simulink model "mcb_pmsm_param_est_MCSPTE1AK144"  (R2023a)
settings: Solver=FixedStepDiscrete  StartTime=0.0  StopTime=6  RelTol=1e-3  EnableMultiTasking=on
PreLoadFcn:
  | mcb_pmsm_param_est_MCSPTE1AK144_data;
InitFcn:
  | mbd_s32k_consistency_checks(bdroot(gcs));
undefined symbols (not defined in the file): External, inverter, LQFP, motor, One, Shot, TRGMUX_PDB_TRIG, Ts, Ts_uart
libraries: mbd_s32k1xx_ec_toolbox x30, simulink x6, mbd_msd_ec_toolbox x4, mcbpmsmparamestlib x4, embeddedblockslib x1
Description:
  | Open Loop Loop Control of 3-phase motor with MTRDEVSPNK144.
  | This Simulink model is designed to work with Linix 45ZWN24-40 Motor and validate
  | that the motor can be rotated in open loop using Mathworks model from Motor Control Blockset.
  | The main scope of the model is to validate the 3-phase current measurements.
  | 
  | FEATURES:
  | - Alternatively, use FreeMASTER pannel to control the speed and direction
  | - Measure the 3-phase sinusoidal currents with PWM-PDB-ADC synchronization
  | - Measure the DC bus voltage and current with PWM-PDB-ADC synchronization
  | 
  | HW SETUP:
  | - Configure S32K144 board supply voltage: J107:2-3(over USB)
  | - Configure J9,J10 and J11 on MotorGD: 2-3 (mode PMSM)
  | - Rotate trimmer resistor R72 (placed Devkit-MotorGD) counter-clockwise at maximum
  | - Power on the kit via J7 connector with 12Vdc
  | 
  | VALIDATION:
  | - First run 'mcb_open_loop_control_data_MTRDEVKSPNK144.m' file to load parameters in workspace,
  | - Build/Simulate the model,
  | - After reset or power on, the Green LED shall be ON
  | - In case of a FAULT the Red LED will be ON
  | - Open FreeMASTER project and connect to the target.
  | - Click on "App" tab and set the desired motor speed then click on the ON/OFF button
  | 
  | NOTE:
  | - In case of fault (RED LED is ON), the remove fault cause and press RESET button
  | 
  | Copyright (c) 2020 NXP
  | version 1.0.0
settings Model: Creator=NXP MBDT Team  LastModifiedBy=snarayan
settings SolverCC: AlgebraicLoopSolver=TrustRegion  AutoInsertRateTranBlk=on
settings DataIOCC: ExternalInput=off  InitialState=off  SaveFormat=Array  SaveOutput=off  SaveTime=off  ReturnWorkspaceOutputs=off
settings OptimizationCC: DefaultParameterBehavior=Inlined  UseFloatMulNetSlope=on  DefaultUnderspecifiedDataType=single  UseSpecifiedMinMax=on  EnhancedBackFolding=on  PassReuseOutputArgsAs=Individual arguments  ZeroExternalMemoryAtStartup=off  ZeroInternalMemoryAtStartup=off  NoFixptDivByZeroProtection=on  EfficientFloat2IntCast=on  OptimizeBlockOrder=speed  DifferentSizesBufferReuse=on  EfficientTunableParamExpr=on
settings DebuggingCC: CheckSSInitialOutputMsg=off  UnderspecifiedInitializationDetection=Classic  MergeDetectMultiDrivingBlocksExec=none  SolverPrmCheckMsg=warning  InheritedTsInSrcMsg=none  MultiTaskDSMMsg=none  SingleTaskRateTransMsg=error  ParameterPrecisionLossMsg=none  ParameterTunabilityLossMsg=error  UnconnectedInputMsg=error  UnconnectedOutputMsg=error  UnconnectedLineMsg=error  AssertControl=DisableAll  AllowSymbolicDim=off  UnknownTsInhSupMsg=error  StateNameClashWarn=warning  SFUnexpectedBacktrackingDiag=warning  SFNoUnconditionalDefaultTransitionDiag=warning  SFExecutionAtInitializationDiag=none  ArithmeticOperatorsInVariantConditions=warning
settings HardwareCC: ProdBitPerPointer=32  ProdBitPerSizeT=32  ProdBitPerPtrDiffT=32  ProdLargestAtomicInteger=Long  ProdLargestAtomicFloat=Double  ProdWordSize=32  ProdHWDeviceType=ARM Compatible->ARM Cortex
settings ModelReferenceCC: EnableRefExpFcnMdlSchedulingChecks=on
settings SFSimCC: SimUseLocalCustomCode=off  MATLABDynamicMemAlloc=off  CustomCodeUndefinedFunction=UseInterfaceOnly
settings RTWCC: Description=Model Based Design Toolbox S32K1xx Code Generation Target  SystemTargetFile=mbd_s32k.tlc  MakeCommand=mbd_s32k_make_rtw COPY_MDLREF_INCLUDES=0  TemplateMakefile=mbd_s32k.tmf  RTWUseLocalCustomCode=off  IncludeHyperlinkInReport=on  DLArmComputeVersion=19.05
settings CodeAppCC: ForceParamTrailComments=on  IgnoreCustomStorageClasses=off  MaxIdLength=64  OperatorAnnotations=on  SimulinkDataObjDesc=on  SFDataObjDesc=on  InsertBlockDesc=on  InternalIdentifier=Classic
settings STFCustomTargetCC: MultiwordLength=256  ConcurrentExecutionCompliant=off  CombineOutputUpdateFcns=on  ERTCustomFileBanners=on  SupportContinuousTime=off  SupportNonInlinedSFcns=off  RemoveResetFunc=on  MATLABClassNameForMDSCustomization=Simulink.SoftwareTarget.ERTCustomization  GRTInterface=off  UseToolchainInfoCompliant=off  SystemTargetFile=mbd_s32k.tlc
settings ERTTargetCC: TargetLangStandard=C99 (ISO)  ParMdlRefBuildCompliant=off  CompOptLevelCompliant=off  ConcurrentExecutionCompliant=off  ModelStepFunctionPrototypeControlCompliant=off  CPPClassGenCompliant=off  UseToolchainInfoCompliant=off  InlinedParameterPlacement=NonHierarchical  ERTSrcFileBannerTemplate=mbd_ert_code_template.cgt  ERTHdrFileBannerTemplate=mbd_ert_code_template.cgt  ERTDataSrcFileTemplate=mbd_ert_code_template.cgt  ERTDataHdrFileTemplate=mbd_ert_code_template.cgt  ERTCustomFileTemplate=example_file_process.tlc
settings ConfigComp: CovMetricSettings=dw  CovSaveCumulativeToWorkspaceVar=on  CovSaveSingleToWorkspaceVar=on  CovExternalEMLEnable=off

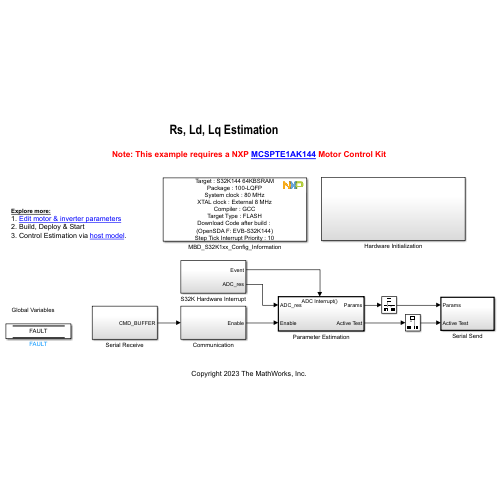
[thumbnail: Simulink's stored preview of the top-level diagram]
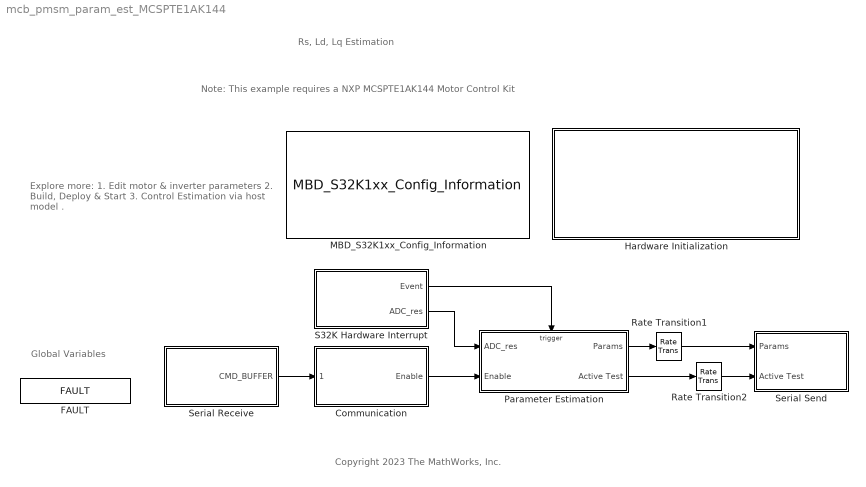
== system mcb_pmsm_param_est_MCSPTE1AK144 ==
  note: Copyright 2023 The MathWorks, Inc.
  note: Rs, Ld, Lq Estimation
  note: Explore more:
      | 1. Edit motor & inverter parameters
      | 2. Build, Deploy & Start
      | 3. Control Estimation via host model .
  note: Note: This example requires a NXP MCSPTE1AK144 Motor Control Kit
  note: Global Variables
  Communication : Subsystem
  FAULT : DataStoreMemory  DataStoreName=FAULT  WriteAfterWriteMsg=warning  WriteAfterReadMsg=warning  ShowAdditionalParam=off  OutDataTypeStr=boolean
  Hardware Initialization : Subsystem  Priority=2
  MBD_S32K1xx_Config_Information : mbd_s32k1xx_ec_toolbox/MBD_S32K1xx_Config_Information  Priority=1  mbdt_ver=0  disp_str=|  config_params=[]  mcu_target_name=S32K144  mcu_target_package=100-LQFP  mcu_target_sram_size=64KB  mcu_system_clock_freq=80  mcu_xtal_freq=External 8  mcu_steptick_timer=LPIT Channel 0  mcu_steptick_prio=10  ds_import_enable=on  target_compiler=GCC  target_memory=FLASH  gcc_target_compile_opts=-mcpu=cortex-m4 -mthumb -mfloat-abi=hard -mfpu=fpv4-sp-d16 -O1 -g -gstrict-dwarf  gcc_target_assemble_opts=-mcpu=cortex-m4 -mthumb -mfloat-abi=hard -mfpu=fpv4-sp-d16 -g  gcc_target_link_opts=-mcpu=cortex-m4 -mthumb -mfloat-abi=hard -mfpu=fpv4-sp-d16  gcc_target_default_lcf=on  gcc_target_user_lcf=S32K144_64_flash.ld  ghs_target_compile_opts=-cpu=cortexm4f -thumb -DARM_MATH_CM4 -fpu=vfpv4_d16 -fsingle -Ogeneral -Wundef -Wimplicit-int -Wshadow -Wtrigraphs --no_commons --gnu_asm -gnu99 -gdwarf-2 -G  ghs_target_assemble_opts=-cpu=cortexm4f -fpu=vfpv4_d16  ghs_target_link_opts=-cpu=cortexm4f -thumb -fpu=vfpv4_d16  ghs_target_default_lcf=on  ghs_target_user_lcf=S32K144_64_flash.ld  iar_target_compile_opts=--cpu=Cortex-M4F --thumb --fpu=VFPv4_sp -Ol -e --debug --dlib_config normal  iar_target_assemble_opts=--cpu Cortex-M4F --thumb --fpu VFPv4_sp  iar_target_link_opts=--no_exceptions --vfe --inline  iar_target_default_lcf=on  iar_target_user_lcf=S32K144_64_flash.icf  pil_download_enable=off  rbl_download_enable=on  rbl_start_delay=5000  rbl_download_interface=OpenSDA  rbl_restart_request=off  rbl_com_port=Custom  rbl_com_port_custom=COM1  pil_download_rate=57600  pil_opensda_drive=F: EVB-S32K144  pil_opensda_drive_custom=D  pil_uart_instance=1  pil_uart_rx=PTC6: [LPUART1_RX | Receive]  pil_uart_tx=PTC7: [LPUART1_TX | Transmit]  FTM_PWM_PcrCheckEnDis=on  FTM_Input_Edge_Inputs_PcrCheckEnDis=on  FTM_Dual_Edge_Inputs_PcrCheckEnDis=on  FTM_Quadrature_Inputs_PcrCheckEnDis=on  FTM_Hall_Sensor_Inputs_PcrCheckEnDis=on  LPTMR_PcrCheckEnDis=on  PIT_PcrCheckEnDis=on  RTC_PcrCheckEnDis=on  FlexCAN_PcrCheckEnDis=on  LIN_PcrCheckEnDis=on  FlexIO_PcrCheckEnDis=on  LPI2C_PcrCheckEnDis=on  LPSPI_PcrCheckEnDis=on  LPUART_PcrCheckEnDis=on  CMP_PcrCheckEnDis=on  GPIO_OutputPcrCheckEnDis=on  GPIO_InputPcrCheckEnDis=on  SBC_PcrCheckEnDis=on  BMS_PcrCheckEnDis=on  AMMCLIB_PcrCheckEnDis=on  FM_PcrCheckEnDis=on  Profile_PcrCheckEnDis=on  ConfigParams_PcrCheckEnDis=on  ModelRef_PcrCheckEnDis=on  PDB0_PcrCheckEnDis=on  CSEc_PcrCheckEnDis=on  eDMA_PcrCheckEnDis=on  FLASH_PcrCheckEnDis=on  ADC_PcrCheckEnDis=on  WDOG_PcrCheckEnDis=on
      | Target : S32K144-64KB_SRAM
      | Package : 100-pin
      | System clock : 80 MHz
      | XTAL clock : External 8 MHz
      | Compiler : IAR
      | Target Type : FLASH
      | Download Code after build : off
      | Step Tick Interrupt Priority : 15
  Parameter Estimation : Subsystem
      settings: RTWSystemCode=Nonreusable function
  Rate Transition1 : RateTransition  Integrity=off  Deterministic=off
  Rate Transition2 : RateTransition  Integrity=off  Deterministic=off
  S32K Hardware Interrupt : Subsystem
  Serial Receive : Subsystem  SystemSampleTime=1e-3
      settings: RTWSystemCode=Nonreusable function
  Serial Send : Subsystem  TreatAsAtomicUnit=on  SystemSampleTime=Ts_uart
  wires:
  Rate Transition1/1 -> Serial Send/1(Params)
  S32K Hardware Interrupt/2(ADC_res) -> Parameter Estimation/1(ADC_res)
  S32K Hardware Interrupt/1(Event) -> Parameter Estimation/Trigger
  Communication/1(Enable) -> Parameter Estimation/2(Enable)
  Serial Receive/1(CMD_BUFFER) -> Communication/1(" ")
  Parameter Estimation/1(Params) -> Rate Transition1/1
  Parameter Estimation/2(Active Test) -> Rate Transition2/1
  Rate Transition2/1 -> Serial Send/2(Active Test)

== system mcb_pmsm_param_est_MCSPTE1AK144/Communication ==
  " " : Inport
  Data Type Conversion : DataTypeConversion  OutDataTypeStr=int16  ConvertRealWorld=Stored Integer (SI)  RndMeth=Simplest  SaturateOnIntegerOverflow=off
  Data Type Conversion3 : DataTypeConversion  OutDataTypeStr=boolean  RndMeth=Simplest  SaturateOnIntegerOverflow=off
  Demux : Demux  Outputs=2
  Rate Transition : RateTransition  Deterministic=off  InitialCondition=[0 0]  OutPortSampleTime=Ts
  Terminator : Terminator
  Enable : Outport  VectorParamsAs1DForOutWhenUnconnected=off
  wires:
  " "/1 -> Rate Transition/1
  Rate Transition/1 -> Demux/1
  Demux/2 -> Data Type Conversion3/1
  Demux/1 -> Data Type Conversion/1
  Data Type Conversion3/1 -> Enable/1
  Data Type Conversion/1 -> Terminator/1

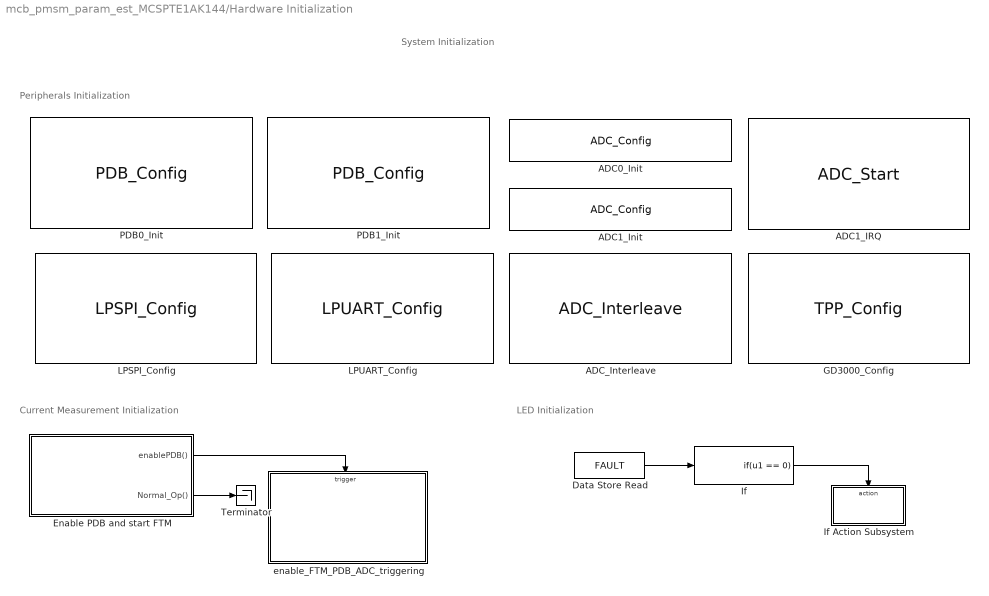
== system mcb_pmsm_param_est_MCSPTE1AK144/Hardware Initialization ==
  note: Peripherals Initialization
  note: System Initialization
  note: Current Measurement Initialization
  note: LED Initialization
  ADC0_Init : mbd_s32k1xx_ec_toolbox/Motor Control Blocks/ADC Blocks/ADC_Config  Priority=3  instance=0  mode=12-bit conversion  smplts=2  adiclk=alternate clock 1  adiv=input clock  show_adv_opts=on  pretrgsel=PDB pre-trigger  swpretrg=Disabled  adtrg=hardware  trgsel=PDB output  refsel=Vrefh and Vrefl  supply_monitoring=off  acfe=off  acfgt=off  acren=off  cv1=0  cv2=0  adco=off  avge=off  avgs=4 samples
  ADC1_IRQ : mbd_s32k1xx_ec_toolbox/Motor Control Blocks/ADC Blocks/ADC_Start  Priority=5  instance=1  adc_r=C  adc_chan=PTB16: [ADC1_SE15 | ADC Single Ended Input]  aien=on  mcuTargetUpdate=on
  ADC1_Init : mbd_s32k1xx_ec_toolbox/Motor Control Blocks/ADC Blocks/ADC_Config  Priority=4  instance=1  mode=12-bit conversion  smplts=2  adiclk=alternate clock 1  adiv=input clock  show_adv_opts=on  pretrgsel=PDB pre-trigger  swpretrg=Disabled  adtrg=hardware  trgsel=PDB output  refsel=Vrefh and Vrefl  supply_monitoring=off  acfe=off  acfgt=off  acren=off  cv1=0  cv2=0  adco=off  avge=off  avgs=4 samples
  ADC_Interleave : mbd_s32k1xx_ec_toolbox/Motor Control Blocks/ADC Blocks/ADC_Interleave  adcInterleavePins=PTB1 to ADC0_SE5 and ADC1_SE15  adcInterleaveInit=on
  Data Store Read : DataStoreRead  DataStoreName=FAULT  IndexOptions=Index vector (dialog)  Indices=1  OutputSizes=1
  Enable PDB and start FTM : Stateflow chart  TreatAsAtomicUnit=on
  GD3000_Config : mbd_msd_ec_toolbox/TPP/TPP_Config  Priority=1  tppInstance=0  desatMode=on  fullonMode=off  lockMode=off  overtempEvent=on  phaseEvent=off  desatEvent=off  framingEvent=on  vlsEvent=on  writeErrEvent=on  overcurrentEvent=on  resetEvent=on  mcuTppIntEn=off  prioInt=15  tppDeadtime=500  initTppNow=on  tppSpiInst=0  tppPwmModule=3  tppPair0_1=on  tppPair2_3=on  tppPair4_5=on  tppPair6_7=off  tppFirstChHS=on  tppEn1Pin=PTA2: [PTA2 | Port A I/O]  tppEn2Pin=PTA2: [PTA2 | Port A I/O]  tppRstPin=PTA3: [PTA3 | Port A I/O]  tppCsPin=PTB5: [PTB5 | Port B I/O]  tppIntPin=PTE10: [PTE10 | Port E I/O]
  If : If  IfExpression=u1 == 0  ShowElse=off
  If Action Subsystem : Subsystem  TreatAsAtomicUnit=on
  "LPSPI_Config " : mbd_s32k1xx_ec_toolbox/Communication Blocks/SPI Blocks/LPSPI_Config   InstanceNumber=0  Role=Master  BaudRate=2000000  ShowAdvanced=on  sin=PTB3: [LPSPI0_SIN | LPSPI Serial Data Input]  sout=PTB4: [LPSPI0_SOUT | LPSPI Serial Data Output]  sck=PTB2: [LPSPI0_SCK | LPSPI Serial Clock I/O]  pcs0=None  pcs1=PTB5: [LPSPI0_PCS1 | Peripheral Chip Select 1]  pcs2=None  pcs3=None  CPHA=1  CPOL=0  BitOrder=MSB first  TransferSize=8  WhichPCS=0  PCSPol=ActiveLow  ContinuousTransfer=off
  LPUART_Config : mbd_s32k1xx_ec_toolbox/Communication Blocks/UART Blocks/LPUART_Config  Priority=1  instance=1  baudrate=256000  databits=8  parity=None  sbns=1  bothedge=rising edge  rxinv=off  txinv=off  show_adv_opts=on  brk13=13 - 16 bit times  lbkde=13 - 16 bit times  rx=PTC6: [LPUART1_RX | Receive]  tx=PTC7: [LPUART1_TX | Transmit]  cts=PTA6: [LPUART1_CTS | Clear To Send (bar)]  rts=PTA7: [LPUART1_RTS | Request To Send]
  PDB0_Init : mbd_s32k1xx_ec_toolbox/Motor Control Blocks/PDB Blocks/PDB_Config  Priority=1  pdbModule=0  regScCont=One-Shot  regScTrgsel=External (TRGMUX_PDB_TRIG)  trgMuxSel=FTM3 Initialize Trigger  trgMuxSelPin=PTB5: [TRGMUX_IN0 | Trigger Mux Input]  regModModulus=5000  regScPrescaler=1  regScMult=1  regPoenPoen0=off  regPo0DlyDly1=0  regPo0DlyDly2=0  enable_pdb_init=off  show_adv_opts=on  regCh0C1En0=on  regCh0C1En1=off  regCh0C1En2=off  regCh0C1En3=off  regCh0C1En4=off  regCh0C1En5=off  regCh0C1En6=off  regCh0C1En7=off  regCh0C1Bb0=off  regCh0C1Bb1=off  regCh0C1Bb2=off  regCh0C1Bb3=off  regCh0C1Bb4=off  regCh0C1Bb5=off  regCh0C1Bb6=off  regCh0C1Bb7=off  regCh0C1Tos0=Pre-trigger is in delay mode  regCh0C1Tos1=Pre-trigger is in delay mode  regCh0C1Tos2=Pre-trigger is in delay mode  regCh0C1Tos3=Pre-trigger is in delay mode  regCh0C1Tos4=Pre-trigger is in delay mode  regCh0C1Tos5=Pre-trigger is in delay mode  regCh0C1Tos6=Pre-trigger is in delay mode  regCh0C1Tos7=Pre-trigger is in delay mode  regCh0DlyDly0=2000  regCh0DlyDly1=0  regCh0DlyDly2=0  regCh0DlyDly3=0  regCh0DlyDly4=0  regCh0DlyDly5=0  regCh0DlyDly6=0  regCh0DlyDly7=0  regCh1C1En0=off  regCh1C1En1=off  regCh1C1En2=off  regCh1C1En3=off  regCh1C1En4=off  regCh1C1En5=off  regCh1C1En6=off  regCh1C1En7=off  regCh1C1Bb0=off  regCh1C1Bb1=off  regCh1C1Bb2=off  regCh1C1Bb3=off  regCh1C1Bb4=off  regCh1C1Bb5=off  regCh1C1Bb6=off  regCh1C1Bb7=off  regCh1C1Tos0=Pre-trigger is in delay mode  regCh1C1Tos1=Pre-trigger is in delay mode  regCh1C1Tos2=Pre-trigger is in delay mode  regCh1C1Tos3=Pre-trigger is in delay mode  regCh1C1Tos4=Pre-trigger is in delay mode  regCh1C1Tos5=Pre-trigger is in delay mode  regCh1C1Tos6=Pre-trigger is in delay mode  regCh1C1Tos7=Pre-trigger is in delay mode  regCh1DlyDly0=0  regCh1DlyDly1=0  regCh1DlyDly2=0  regCh1DlyDly3=0  regCh1DlyDly4=0  regCh1DlyDly5=0  regCh1DlyDly6=0  regCh1DlyDly7=0
  PDB1_Init : mbd_s32k1xx_ec_toolbox/Motor Control Blocks/PDB Blocks/PDB_Config  Priority=2  pdbModule=1  regScCont=One-Shot  regScTrgsel=External (TRGMUX_PDB_TRIG)  trgMuxSel=FTM3 Initialize Trigger  trgMuxSelPin=PTB5: [TRGMUX_IN0 | Trigger Mux Input]  regModModulus=5000  regScPrescaler=1  regScMult=1  regPoenPoen0=off  regPo0DlyDly1=0  regPo0DlyDly2=0  enable_pdb_init=off  show_adv_opts=on  regCh0C1En0=on  regCh0C1En1=on  regCh0C1En2=on  regCh0C1En3=off  regCh0C1En4=off  regCh0C1En5=off  regCh0C1En6=off  regCh0C1En7=off  regCh0C1Bb0=off  regCh0C1Bb1=off  regCh0C1Bb2=off  regCh0C1Bb3=off  regCh0C1Bb4=off  regCh0C1Bb5=off  regCh0C1Bb6=off  regCh0C1Bb7=off  regCh0C1Tos0=Pre-trigger is in delay mode  regCh0C1Tos1=Pre-trigger is in delay mode  regCh0C1Tos2=Pre-trigger is in delay mode  regCh0C1Tos3=Pre-trigger is in delay mode  regCh0C1Tos4=Pre-trigger is in delay mode  regCh0C1Tos5=Pre-trigger is in delay mode  regCh0C1Tos6=Pre-trigger is in delay mode  regCh0C1Tos7=Pre-trigger is in delay mode  regCh0DlyDly0=0  regCh0DlyDly1=1000  regCh0DlyDly2=2000  regCh0DlyDly3=0  regCh0DlyDly4=0  regCh0DlyDly5=0  regCh0DlyDly6=0  regCh0DlyDly7=0  regCh1C1En0=off  regCh1C1En1=off  regCh1C1En2=off  regCh1C1En3=off  regCh1C1En4=off  regCh1C1En5=off  regCh1C1En6=off  regCh1C1En7=off  regCh1C1Bb0=off  regCh1C1Bb1=off  regCh1C1Bb2=off  regCh1C1Bb3=off  regCh1C1Bb4=off  regCh1C1Bb5=off  regCh1C1Bb6=off  regCh1C1Bb7=off  regCh1C1Tos0=Pre-trigger is in delay mode  regCh1C1Tos1=Pre-trigger is in delay mode  regCh1C1Tos2=Pre-trigger is in delay mode  regCh1C1Tos3=Pre-trigger is in delay mode  regCh1C1Tos4=Pre-trigger is in delay mode  regCh1C1Tos5=Pre-trigger is in delay mode  regCh1C1Tos6=Pre-trigger is in delay mode  regCh1C1Tos7=Pre-trigger is in delay mode  regCh1DlyDly0=0  regCh1DlyDly1=0  regCh1DlyDly2=0  regCh1DlyDly3=0  regCh1DlyDly4=0  regCh1DlyDly5=0  regCh1DlyDly6=0  regCh1DlyDly7=0
  Terminator : Terminator
  enable_FTM_PDB_ADC_triggering : Subsystem  TreatAsAtomicUnit=on
      settings: RTWSystemCode=Inline
  wires:
  Enable PDB and start FTM/1(enablePDB()) -> enable_FTM_PDB_ADC_triggering/Trigger
  Enable PDB and start FTM/2(Normal_Op()) -> Terminator/1
  Data Store Read/1 -> If/1
  If/1 -> If Action Subsystem/Action

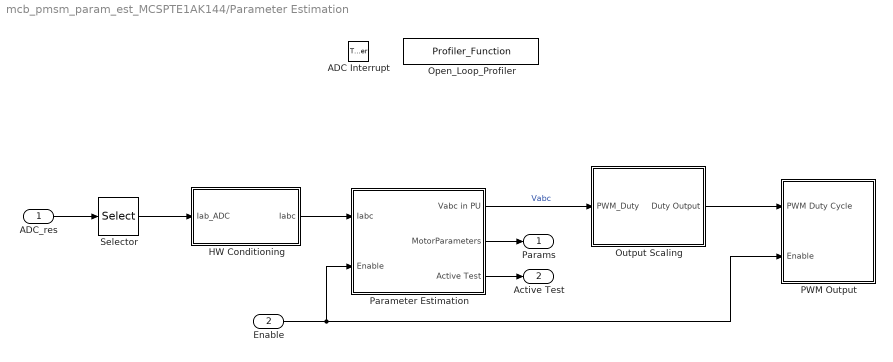
== system mcb_pmsm_param_est_MCSPTE1AK144/Parameter Estimation ==
  ADC_res : Inport
  Enable : Inport  Port=2
  ADC Interrupt : TriggerPort  TriggerType=function-call  VariantControl=Variant
  HW Conditioning : Subsystem
  Open_Loop_Profiler : mbd_s32k1xx_ec_toolbox/Utility Blocks/Profiler_Function  profile_indx=1
  Output Scaling : Subsystem
  PWM Output : Subsystem
  Parameter Estimation : Subsystem
  Selector : Selector  InputPortWidth=4  IndexOptions=Index vector (dialog)  Indices=[1 2]  OutputSizes=1
  Params : Outport
  Active Test : Outport  Port=2
  wires:
  ADC_res/1 -> Selector/1
  Parameter Estimation/1(Vabc in PU) -> Output Scaling/1(PWM_Duty)  "Vabc"
  Output Scaling/1(Duty Output) -> PWM Output/1(PWM Duty Cycle)
  Enable/1 -> Parameter Estimation/2(Enable), PWM Output/2(Enable)
  Parameter Estimation/2(MotorParameters) -> Params/1
  HW Conditioning/1(Iabc) -> Parameter Estimation/1(Iabc)
  Selector/1 -> HW Conditioning/1(Iab_ADC)
  Parameter Estimation/3(Active Test) -> Active Test/1

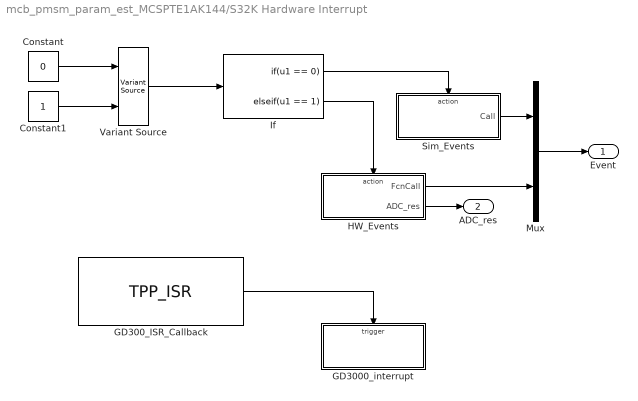
== system mcb_pmsm_param_est_MCSPTE1AK144/S32K Hardware Interrupt ==
  Constant : Constant  Value=0  OutDataTypeStr=Inherit: Inherit via back propagation  SampleTime=-1
  Constant1 : Constant  OutDataTypeStr=Inherit: Inherit via back propagation  SampleTime=-1
  GD3000_interrupt : Subsystem  TreatAsAtomicUnit=on
  "GD300_ISR_Callback " : mbd_msd_ec_toolbox/TPP/TPP_ISR  tppInstance=0
  HW_Events : Subsystem  TreatAsAtomicUnit=on
  If : If  IfExpression=u1 == 0  ElseIfExpressions=u1 == 1  ShowElse=off
  Mux : Mux  Inputs=2
  Sim_Events : Subsystem  TreatAsAtomicUnit=on
  Variant Source : VariantSource  VariantControlMode=sim codegen switching
  Event : Outport
  ADC_res : Outport  Port=2
  wires:
  Constant/1 -> Variant Source/1
  Constant1/1 -> Variant Source/2
  If/2 -> HW_Events/Action
  If/1 -> Sim_Events/Action
  Variant Source/1 -> If/1
  Sim_Events/1(Call) -> Mux/1
  HW_Events/1(FcnCall) -> Mux/2
  Mux/1 -> Event/1
  "GD300_ISR_Callback "/1 -> GD3000_interrupt/Trigger
  HW_Events/2(ADC_res) -> ADC_res/1

== system mcb_pmsm_param_est_MCSPTE1AK144/Serial Receive ==
  Codegen : Subsystem
  Sim : Subsystem
  Variant Source : VariantSource  VariantControlMode=sim codegen switching
  CMD_BUFFER : Outport  InitialOutput=[16384 0]  VectorParamsAs1DForOutWhenUnconnected=off
  wires:
  Sim/1(Out1) -> Variant Source/2
  Variant Source/1 -> CMD_BUFFER/1
  Codegen/1(Out1) -> Variant Source/1

== system mcb_pmsm_param_est_MCSPTE1AK144/Serial Send ==
  Params : Inport
  Active Test : Inport  Port=2
  Demux : Demux  Outputs=3
  LPUART_Transmit : mbd_s32k1xx_ec_toolbox/Communication Blocks/UART Blocks/LPUART_Transmit  Priority=2  instance=1
  Multiport Switch : MultiPortSwitch  DiagnosticForDefault=Warning  OutDataTypeStr=dataType  RndMeth=Simplest  SaturateOnIntegerOverflow=off  InputSameDT=off
  Protocol Encoder : embeddedblockslib/Protocol Encoder  Header='S'  FieldTable={ 'Count', '1', 'uint8', 'Little endian'; 'Parameter', '1', 'single', 'Little endian'; 'Active Test', '1', 'uint8', 'Little endian' }  IsChecksumRequired=off  ChecksumAlgorithm=XOR of bytes  ChecksumSize=[]  TerminatorOption=<none>  CustomTerminatorVal=[]
      settings: LibrarySourceBlock=c2000lib/Target Communication/Protocol Encoder
  Reshape : Reshape
  count to 3 : Subsystem
  wires:
  Protocol Encoder/1 -> Reshape/1
  Reshape/1 -> LPUART_Transmit/1
  Multiport Switch/1 -> Protocol Encoder/2
  Params/1 -> Demux/1
  Demux/1 -> Multiport Switch/2
  Demux/2 -> Multiport Switch/3
  Demux/3 -> Multiport Switch/4
  count to 3/1(count) -> Multiport Switch/1, Protocol Encoder/1
  Active Test/1 -> Protocol Encoder/3

== system mcb_pmsm_param_est_MCSPTE1AK144/Hardware Initialization/If Action Subsystem ==
  Action Port : ActionPort  ActionPortLabel=if(u1 == 0)
  LED_GREEN : Constant  Value=0  OutDataTypeStr=boolean  SampleTime=-1
  LED_GREEN_ON : mbd_s32k1xx_ec_toolbox/GPIO Blocks/Digital_Output  gpio_pin=PTD16: [PTD16 | Port D I/O]  init_val=Low  drive_strength=Low
  LED_RED : Constant  OutDataTypeStr=boolean  SampleTime=-1
  LED_RED_OFF : mbd_s32k1xx_ec_toolbox/GPIO Blocks/Digital_Output  gpio_pin=PTD15: [PTD15 | Port D I/O]  init_val=Low  drive_strength=Low
  wires:
  LED_GREEN/1 -> LED_GREEN_ON/1
  LED_RED/1 -> LED_RED_OFF/1

== system mcb_pmsm_param_est_MCSPTE1AK144/Hardware Initialization/enable_FTM_PDB_ADC_triggering ==
  function : TriggerPort  TriggerType=function-call  VariantControl=(inherit)
  Custom code to reload the PDB value : Subsystem  Priority=6  mask(System Outputs){ShowInLibBrowser=0}
      mask prompts: ShowInLibBrowser "Simulink:masks:CustCodeMaskParam1_MP"
      settings: CopyFcn=cccopyfcn(gcb)  OpenFcn=ccopenfcn('System Outputs Function')
      mask Help: eval('feval(''rtwprivate'',''rtwhelpview'',''rtw_sys_outputs_block'')');
      mask Display: disp('System\nOutputs');
  FTM_Init_Trigger_Disable_Enable : mbd_s32k1xx_ec_toolbox/Motor Control Blocks/FTM Blocks/FTM_Init_Trigger_Disable_Enable  Priority=3  ftmModule=3  action=Enable
  FTM_PWM_Disable_Enable : mbd_s32k1xx_ec_toolbox/Motor Control Blocks/FTM Blocks/FTM_PWM_Disable_Enable  Priority=1  ftmModule=3  action=Enable
  PDB0_Enable : mbd_s32k1xx_ec_toolbox/Motor Control Blocks/PDB Blocks/PDB_Enable  Priority=4  pdbModule=0  pdbAction=Enable
  PDB1_Enable : mbd_s32k1xx_ec_toolbox/Motor Control Blocks/PDB Blocks/PDB_Enable  Priority=5  pdbModule=1  pdbAction=Enable
  TPP_ISR_Enable_Disable : mbd_msd_ec_toolbox/TPP/TPP_ISR_Enable_Disable  Priority=7  tppInstance=0  mcuTppIntEn=on  prioInt=15

== system mcb_pmsm_param_est_MCSPTE1AK144/Parameter Estimation/HW Conditioning ==
  Iab_ADC : Inport
  Add : Sum  Inputs=+-  RndMeth=Simplest  OutDataTypeStr=Inherit: Same as first input
  Constant2 : Constant  Value=0  OutDataTypeStr=single
  Data Type Conversion : DataTypeConversion  OutDataTypeStr=single  RndMeth=Simplest  SaturateOnIntegerOverflow=off
  Gain : Gain  Gain=-inverter.ISenseMax/2048  RndMeth=Simplest  OutDataTypeStr=Inherit: Same as input
  Iab Offset : Constant  Value=[inverter.CtSensAOffset inverter.CtSensBOffset]  OutDataTypeStr=int32
  Mux : Mux  Inputs=2
  Iabc : Outport
  wires:
  Add/1 -> Gain/1
  Data Type Conversion/1 -> Add/1
  Iab_ADC/1 -> Data Type Conversion/1
  Iab Offset/1 -> Add/2
  Constant2/1 -> Mux/2
  Mux/1 -> Iabc/1
  Gain/1 -> Mux/1

== system mcb_pmsm_param_est_MCSPTE1AK144/Parameter Estimation/Output Scaling ==
  PWM_Duty : Inport
  Constant : Constant  OutDataTypeStr=dataType
  Gain : Gain  Gain=0.5  RndMeth=Simplest  OutDataTypeStr=Inherit: Same as input
  Sum : Sum  Inputs=|++  RndMeth=Simplest  OutDataTypeStr=Inherit: Same as first input
  Duty Output : Outport
  wires:
  Gain/1 -> Duty Output/1
  PWM_Duty/1 -> Sum/1
  Constant/1 -> Sum/2
  Sum/1 -> Gain/1

== system mcb_pmsm_param_est_MCSPTE1AK144/Parameter Estimation/PWM Output ==
  PWM Duty Cycle : Inport
  Enable : Inport  Port=2
  Demux : Demux  Outputs=3
  FTM_PWM_Config : mbd_s32k1xx_ec_toolbox/Motor Control Blocks/FTM Blocks/FTM_PWM_Config  ftmModule=3  ftmMode=Center-Aligned PWM  ftmSourceClock=80 MHz  swcontrol_enable=off  chan0En=on  chan0Type=Independent  chan2En=on  chan2Type=Independent  chan4En=on  chan4Type=Independent  chan6En=off  chan6Type=Independent  ftmPwmUnits=Hz  outFrequency=20000  ftmPeriod=4000  ftmPrescaler=Divide by 1  deadtimeUnits=Nanoseconds  deadtimeNs=0  deadtimeTicks=0  deadtimePrescaler=Divide by 1  dutyCycleCh0=0  dutyCycleCh1=0  dutyCycleCh2=0  dutyCycleCh3=0  dutyCycleCh4=0  dutyCycleCh5=0  dutyCycleCh6=0.25  dutyCycleCh7=0.25  dutyCycleSim=on  startAfterInit=off  showAdvOpt=on  pinFtmCh0=PTB8: [FTM3_CH0 | FTM Channel]  pinFtmCh1=PTB9: [FTM3_CH1 | FTM Channel]  pinPolCh0=Active Low  pinPolCh1=Active Low  outputComplem0=Main duplicated  outputLevel0=Low  outputLevel1=Low  pinFtmCh2=PTB10: [FTM3_CH2 | FTM Channel]  pinFtmCh3=PTB11: [FTM3_CH3 | FTM Channel]  pinPolCh2=Active Low  pinPolCh3=Active Low  outputComplem2=Main duplicated  outputLevel2=Low  outputLevel3=Low  pinFtmCh4=PTC10: [FTM3_CH4 | FTM Channel]  pinFtmCh5=PTC11: [FTM3_CH5 | FTM Channel]  pinPolCh4=Active Low  pinPolCh5=Active Low  outputComplem4=Main duplicated  outputLevel4=Low  outputLevel5=Low  pinFtmCh6=PTC12: [FTM3_CH6 | FTM Channel]  pinFtmCh7=None  pinPolCh6=Active Low  pinPolCh7=Active Low  outputComplem6=Main duplicated  outputLevel6=Low  outputLevel7=Low  initTrigger=off  chTrigger0=off  chTrigger1=off  chTrigger2=off  chTrigger3=off  chTrigger4=off  chTrigger5=off  chTrigger6=off  chTrigger7=off  mcuTargetUpdate=on  pwmSyncTrg=Software trigger  pwmSyncHwRouting=TRGMUX_FTM7  pwmSyncTrg0=off  pwmSyncTrg1=off  pwmSyncTrg2=off  pwmSyncAutoClear=off  pwmSyncMinLoad=off  pwmSyncMaxLoad=on  pwmSyncInvert=PWM Syncronization  pwmSyncOutControl=PWM Syncronization  pwmSyncOutMask=PWM Syncronization  pwmSyncCounterInitial=PWM Syncronization  pwmSyncPoints=Wait Loading Points  reloadEnable=off  reloadPriority=15  reloadHalfCycle=off  reloadHCR=0  reloadFrequency=0  chnMatch0=off  chnMatch1=off  chnMatch2=off  chnMatch3=off  chnMatch4=off  chnMatch5=off  chnMatch6=off  chnMatch7=off  pwmFaultProtection=off  pwmFaultInterrupt=off  pwmFaultClearing=Fault control disabled  pwmFaultPinState=Safe Value  pwmFaultFilterValue=0  pwmFaultPriority=15  fault_disen_0=off  fault_filter_0=off  fault_polarity_0=Active High  fault_disen_1=off  fault_filter_1=off  fault_polarity_1=Active high  fault_disen_2=off  fault_filter_2=off  fault_polarity_2=Active high  fault_disen_3=off  fault_filter_3=off  fault_polarity_3=Active high  fault_pin_0=None  fault_pin_1=None  fault_pin_2=None  fault_pin_3=None
  Mux2 : Mux  Inputs=3
  Sim PWMs : Scope  NumInputPorts=6
  Switch4 : Switch  Threshold=0.5  RndMeth=Simplest  SaturateOnIntegerOverflow=off  InputSameDT=off
  stop : Constant  Value=0  OutDataTypeStr=dataType
  wires:
  PWM Duty Cycle/1 -> Switch4/1
  stop/1 -> Mux2/3, Mux2/2, Mux2/1
  Mux2/1 -> Switch4/3
  Switch4/1 -> Demux/1
  Enable/1 -> Switch4/2
  FTM_PWM_Config/1 -> Sim PWMs/1
  FTM_PWM_Config/2 -> Sim PWMs/2
  FTM_PWM_Config/3 -> Sim PWMs/3
  FTM_PWM_Config/4 -> Sim PWMs/4
  FTM_PWM_Config/5 -> Sim PWMs/5
  FTM_PWM_Config/6 -> Sim PWMs/6
  Demux/1 -> FTM_PWM_Config/2, FTM_PWM_Config/1  "PWM_A"
  Demux/3 -> FTM_PWM_Config/5, FTM_PWM_Config/6  "PWM_C"
  Demux/2 -> FTM_PWM_Config/4, FTM_PWM_Config/3  "PWM_B"

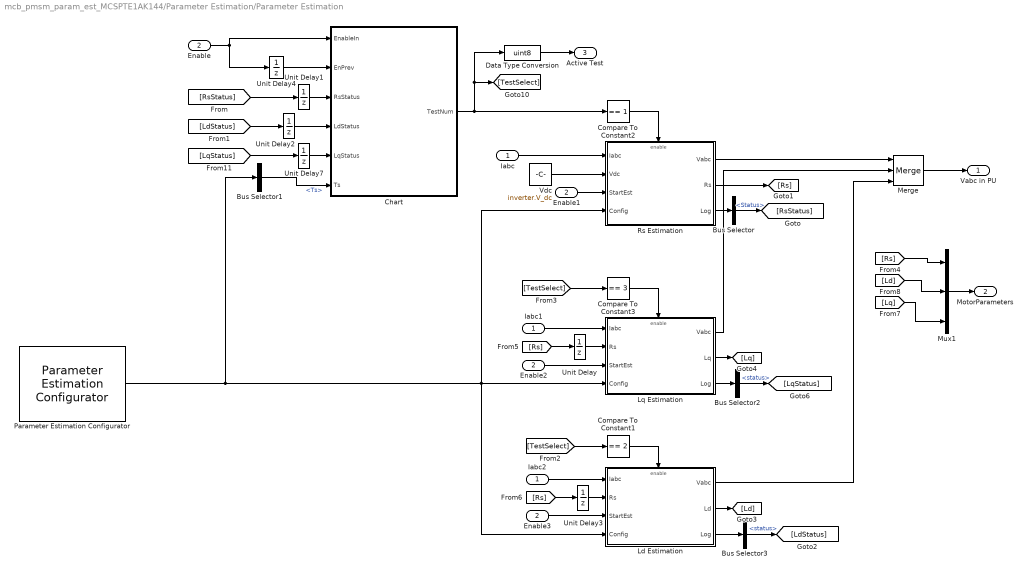
== system mcb_pmsm_param_est_MCSPTE1AK144/Parameter Estimation/Parameter Estimation ==
  Iabc : Inport
  Enable : Inport  Port=2
  Bus Selector : BusSelector  OutputSignals=Status
  Bus Selector1 : BusSelector  OutputSignals=Ts
  Bus Selector2 : BusSelector  OutputSignals=status
  Bus Selector3 : BusSelector  OutputSignals=status
  Chart : Stateflow chart  TreatAsAtomicUnit=on
  Compare To Constant1 : simulink/Logic and Bit Operations/Compare To Constant  relop===  const=2  OutDataTypeStr=boolean
  Compare To Constant2 : simulink/Logic and Bit Operations/Compare To Constant  relop===  const=1  OutDataTypeStr=boolean
  Compare To Constant3 : simulink/Logic and Bit Operations/Compare To Constant  relop===  const=3  OutDataTypeStr=boolean
  Data Type Conversion : DataTypeConversion  OutDataTypeStr=uint8  RndMeth=Simplest  SaturateOnIntegerOverflow=off
  Enable1 : InportShadow  Port=2
  Enable2 : InportShadow  Port=2
  Enable3 : InportShadow  Port=2
  Iabc1 : InportShadow
  Iabc2 : InportShadow
  Ld Estimation : Subsystem
  Lq Estimation : Subsystem
  Merge : Merge  Inputs=3
  Mux1 : Mux  Inputs=3
  Parameter Estimation Configurator : mcbpmsmparamestlib/Parameter Estimation Configurator  P=motor.polePairs  NRated=motor.base_speed  IRated=2.3  ImaxInverter=15.625  RBoard=0.0043  ISenseGain=0.0105  VSenseGain=0.0098  RsTime=2  RsVdRef=0.4  FreqMax=1000  FreqMin=400  FreqStepSweep=100  FreqStepEst=10  FreqNum=10  LdqRotorAlignTime=1  VdqSinePeaktoNeutral=0.2  VdqDCBias=0.4  KeTime=5  KeSpeed=motor.base_speed*0.6  IqRefFOC=0.2  KpKiInputEnable=off  Kp=1  Ki=1000  JSpeedLow=motor.base_speed*0.2  DataType=single  Ts=Ts
      settings: LibrarySourceBlock=mcblib/Parameter Estimation/PMSM Parameter Estimation/Parameter Estimation Configurator
  Rs Estimation : Subsystem
  Unit Delay{,1..4,7} (6 alike) : UnitDelay  SampleTime=-1  HasFrameUpgradeWarning=on
  Vdc : Constant  Value=inverter.V_dc  OutDataTypeStr=single
  Vabc in PU : Outport  VectorParamsAs1DForOutWhenUnconnected=off
  MotorParameters : Outport  Port=2
  Active Test : Outport  Port=3
  wires:
  Parameter Estimation Configurator/1 -> Bus Selector1/1, Ld Estimation/4(Config), Lq Estimation/4(Config), Rs Estimation/4(Config)
  Bus Selector1/1 -> Chart/6(Ts)  "<Ts>"
  Enable/1 -> Unit Delay4/1, Chart/1(EnableIn)
  Bus Selector/1 -> [RsStatus]  "<Status>"
  Bus Selector3/1 -> [LdStatus]  "<status>"
  [RsStatus] -> Unit Delay1/1
  Unit Delay1/1 -> Chart/3(RsStatus)
  [LdStatus] -> Unit Delay2/1
  Unit Delay2/1 -> Chart/4(LdStatus)
  Merge/1 -> Vabc in PU/1
  Vdc/1 -> Rs Estimation/2(Vdc)
  Enable1/1 -> Rs Estimation/3(StartEst)
  Rs Estimation/1(Vabc) -> Merge/1
  Rs Estimation/3(Log) -> Bus Selector/1
  Enable2/1 -> Lq Estimation/3(StartEst)
  Lq Estimation/1(Vabc) -> Merge/2
  Lq Estimation/3(Log) -> Bus Selector2/1
  Enable3/1 -> Ld Estimation/3(StartEst)
  Ld Estimation/1(Vabc) -> Merge/3
  Ld Estimation/3(Log) -> Bus Selector3/1
  Chart/1(TestNum) -> Data Type Conversion/1, [TestSelect], Compare To Constant2/1
  Compare To Constant2/1 -> Rs Estimation/Enable
  [TestSelect] -> Compare To Constant1/1
  Compare To Constant1/1 -> Ld Estimation/Enable
  [TestSelect] -> Compare To Constant3/1
  Compare To Constant3/1 -> Lq Estimation/Enable
  Unit Delay4/1 -> Chart/2(EnPrev)
  Mux1/1 -> MotorParameters/1
  Data Type Conversion/1 -> Active Test/1
  Iabc/1 -> Rs Estimation/1(Iabc)
  Iabc1/1 -> Lq Estimation/1(Iabc)
  Iabc2/1 -> Ld Estimation/1(Iabc)
  Rs Estimation/2(Rs) -> [Rs]
  [Rs] -> Mux1/1
  [Rs] -> Unit Delay/1
  [Rs] -> Unit Delay3/1
  Ld Estimation/2(Ld) -> [Ld]
  Lq Estimation/2(Lq) -> [Lq]
  [Lq] -> Mux1/3
  [Ld] -> Mux1/2
  Unit Delay/1 -> Lq Estimation/2(Rs)
  Unit Delay3/1 -> Ld Estimation/2(Rs)
  Bus Selector2/1 -> [LqStatus]  "<status>"
  Unit Delay7/1 -> Chart/5(LqStatus)
  [LqStatus] -> Unit Delay7/1

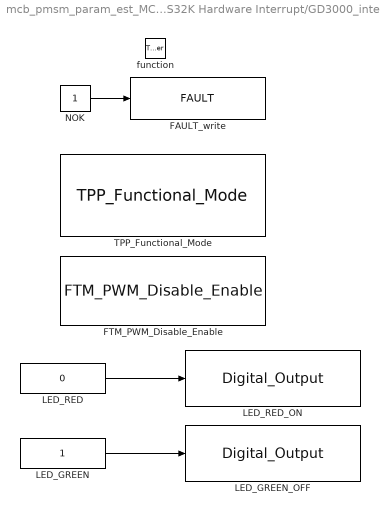
== system mcb_pmsm_param_est_MCSPTE1AK144/S32K Hardware Interrupt/GD3000_interrupt ==
  function : TriggerPort  TriggerType=function-call  VariantControl=Variant
  FAULT_write : DataStoreWrite  DataStoreName=FAULT  IndexOptions=Index vector (dialog)  Indices=1  OutputSizes=1
  FTM_PWM_Disable_Enable : mbd_s32k1xx_ec_toolbox/Motor Control Blocks/FTM Blocks/FTM_PWM_Disable_Enable  ftmModule=3  action=Disable
  LED_GREEN : Constant  OutDataTypeStr=boolean  SampleTime=-1
  LED_GREEN_OFF : mbd_s32k1xx_ec_toolbox/GPIO Blocks/Digital_Output  gpio_pin=PTD16: [PTD16 | Port D I/O]  init_val=Low  drive_strength=Low
  LED_RED : Constant  Value=0  OutDataTypeStr=boolean  SampleTime=-1
  LED_RED_ON : mbd_s32k1xx_ec_toolbox/GPIO Blocks/Digital_Output  gpio_pin=PTD15: [PTD15 | Port D I/O]  init_val=Low  drive_strength=Low
  NOK : Constant  OutDataTypeStr=boolean
  TPP_Functional_Mode : mbd_msd_ec_toolbox/TPP/TPP_Functional_Mode  tppInstance=0  action=Sleep
  wires:
  NOK/1 -> FAULT_write/1
  LED_GREEN/1 -> LED_GREEN_OFF/1
  LED_RED/1 -> LED_RED_ON/1

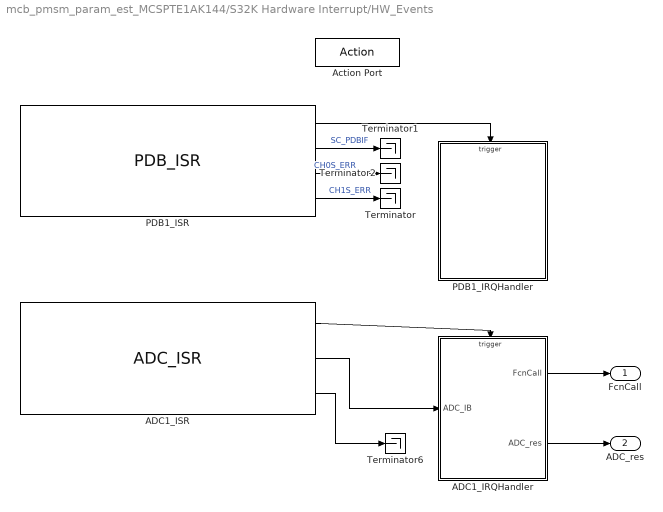
== system mcb_pmsm_param_est_MCSPTE1AK144/S32K Hardware Interrupt/HW_Events ==
  Action Port : ActionPort  ActionPortLabel=elseif(u1 == 1)
  ADC1_IRQHandler : Subsystem  TreatAsAtomicUnit=on
  ADC1_ISR : mbd_s32k1xx_ec_toolbox/Motor Control Blocks/ADC Blocks/ADC_ISR  instance=1  pri=1  sc1n=C
  PDB1_IRQHandler : Subsystem  TreatAsAtomicUnit=on
  PDB1_ISR : mbd_s32k1xx_ec_toolbox/Motor Control Blocks/PDB Blocks/PDB_ISR  Priority=8  pdbModule=1  prioInterrupt=2  regScPdbie=on  regScPdbeie=off  regIdlyIdly=4999
  Terminator{,1..2,6} (4 alike) : Terminator
  FcnCall : Outport  VectorParamsAs1DForOutWhenUnconnected=off
  ADC_res : Outport  Port=2  VectorParamsAs1DForOutWhenUnconnected=off
  wires:
  ADC1_ISR/3 -> Terminator6/1
  ADC1_IRQHandler/1(FcnCall) -> FcnCall/1
  ADC1_ISR/1 -> ADC1_IRQHandler/Trigger
  PDB1_ISR/3 -> Terminator2/1  "CH0S_ERR"
  PDB1_ISR/4 -> Terminator/1  "CH1S_ERR"
  ADC1_ISR/2 -> ADC1_IRQHandler/1(ADC_IB)
  PDB1_ISR/2 -> Terminator1/1  "SC_PDBIF"
  PDB1_ISR/1 -> PDB1_IRQHandler/Trigger
  ADC1_IRQHandler/2(ADC_res) -> ADC_res/1

== system mcb_pmsm_param_est_MCSPTE1AK144/S32K Hardware Interrupt/Sim_Events ==
  Action Port : ActionPort  ActionPortLabel=if(u1 == 0)
  Function-Call Generator : simulink/Ports & Subsystems/Function-Call Generator  sample_time=Ts  numberOfIterations=1  DisallowWideOutput=off
  Call : Outport  VectorParamsAs1DForOutWhenUnconnected=off
  wires:
  Function-Call Generator/1 -> Call/1

== system mcb_pmsm_param_est_MCSPTE1AK144/Serial Receive/Codegen ==
  Constant : Constant  Value=3  OutDataTypeStr=Inherit: Inherit via back propagation
  LPUART_Receive : mbd_s32k1xx_ec_toolbox/Communication Blocks/UART Blocks/LPUART_Receive  instance=1
  Mux2 : Mux  Inputs=2
  Subsystem : Subsystem
  Out1 : Outport
  wires:
  Constant/1 -> LPUART_Receive/1
  Subsystem/2(Out2) -> Mux2/2
  Subsystem/1(Out1) -> Mux2/1
  LPUART_Receive/1 -> Subsystem/1(Input)
  Mux2/1 -> Out1/1

== system mcb_pmsm_param_est_MCSPTE1AK144/Serial Receive/Sim ==
  Constant : Constant  OutDataTypeStr=dataType
  Data Type Conversion : DataTypeConversion  OutDataTypeStr=int16  RndMeth=Simplest  SaturateOnIntegerOverflow=off
  Mux : Mux  Inputs=2
  Speed_ref_rpm (sim) : Constant  Value=600  OutDataTypeStr=dataType  SampleTime=-1
  Out1 : Outport
  wires:
  Speed_ref_rpm (sim)/1 -> Mux/1
  Constant/1 -> Mux/2
  Data Type Conversion/1 -> Out1/1
  Mux/1 -> Data Type Conversion/1

== system mcb_pmsm_param_est_MCSPTE1AK144/Serial Send/count to 3 ==
  Add : Sum  OutDataTypeStr=Inherit: Same as first input
  Constant : Constant  OutDataTypeStr=uint8  SampleTime=-1
  Constant1 : Constant  Value=0  OutDataTypeStr=uint8
  Switch : Switch  Threshold=3  SaturateOnIntegerOverflow=off  InputSameDT=off
  Unit Delay : UnitDelay  SampleTime=-1  HasFrameUpgradeWarning=on
  count : Outport
  wires:
  Switch/1 -> Unit Delay/1
  Constant/1 -> Add/1
  Add/1 -> Switch/3, Switch/2, count/1
  Unit Delay/1 -> Add/2
  Constant1/1 -> Switch/1

== system mcb_pmsm_param_est_MCSPTE1AK144/Hardware Initialization/enable_FTM_PDB_ADC_triggering/Custom code to reload the PDB value ==

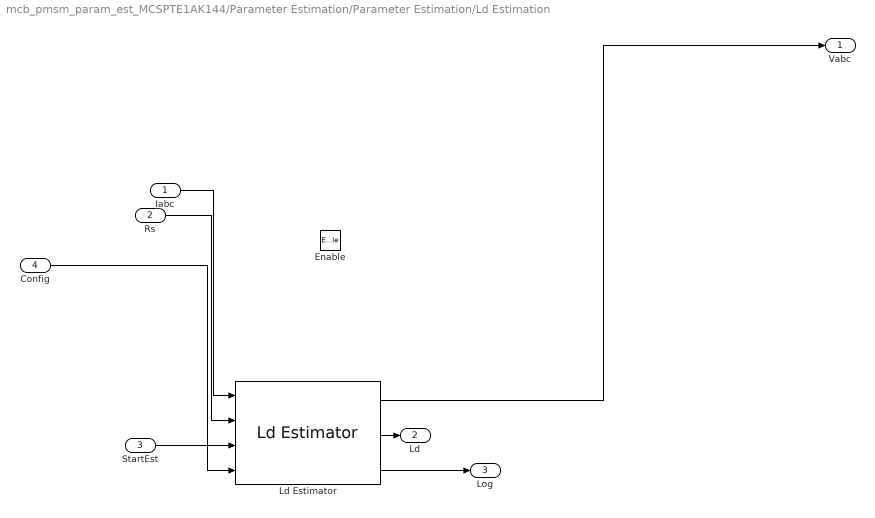
== system mcb_pmsm_param_est_MCSPTE1AK144/Parameter Estimation/Parameter Estimation/Ld Estimation ==
  Iabc : Inport
  Rs : Inport  Port=2
  StartEst : Inport  Port=3
  Config : Inport  Port=4
  Enable : EnablePort  StatesWhenEnabling=reset
  Ld Estimator : mcbpmsmparamestlib/Ld Estimator
  Vabc : Outport
  Ld : Outport  Port=2
  Log : Outport  Port=3
  wires:
  StartEst/1 -> Ld Estimator/3
  Ld Estimator/1 -> Vabc/1
  Iabc/1 -> Ld Estimator/1
  Ld Estimator/3 -> Log/1
  Rs/1 -> Ld Estimator/2
  Ld Estimator/2 -> Ld/1
  Config/1 -> Ld Estimator/4

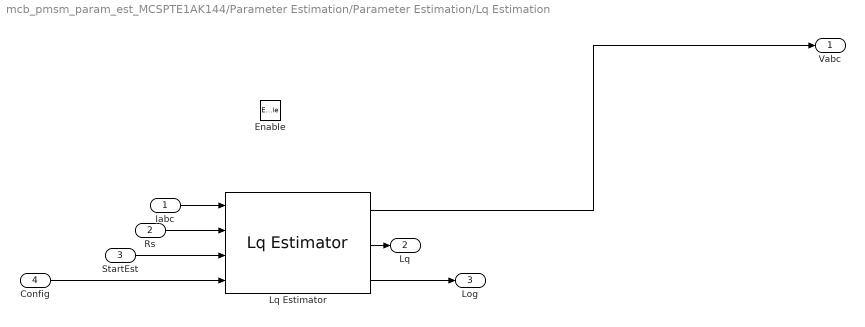
== system mcb_pmsm_param_est_MCSPTE1AK144/Parameter Estimation/Parameter Estimation/Lq Estimation ==
  Iabc : Inport
  Rs : Inport  Port=2
  StartEst : Inport  Port=3
  Config : Inport  Port=4
  Enable : EnablePort  StatesWhenEnabling=reset
  Lq Estimator : mcbpmsmparamestlib/Lq Estimator
      settings: LibrarySourceBlock=mcblib/Parameter Estimation/PMSM Parameter Estimation/Lq Estimator
  Vabc : Outport
  Lq : Outport  Port=2
  Log : Outport  Port=3
  wires:
  Lq Estimator/2 -> Lq/1
  Iabc/1 -> Lq Estimator/1
  Lq Estimator/3 -> Log/1
  StartEst/1 -> Lq Estimator/3
  Lq Estimator/1 -> Vabc/1
  Config/1 -> Lq Estimator/4
  Rs/1 -> Lq Estimator/2

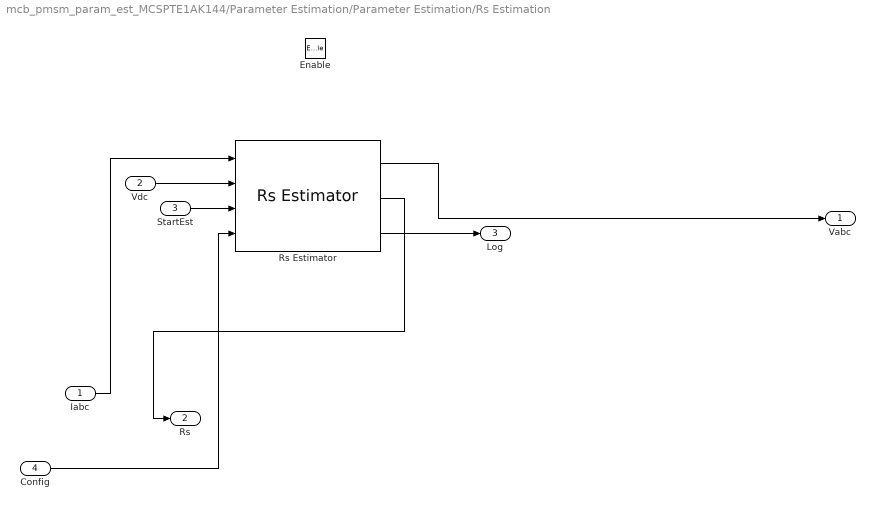
== system mcb_pmsm_param_est_MCSPTE1AK144/Parameter Estimation/Parameter Estimation/Rs Estimation ==
  Iabc : Inport
  Vdc : Inport  Port=2
  StartEst : Inport  Port=3
  Config : Inport  Port=4
  Enable : EnablePort  StatesWhenEnabling=reset
  Rs Estimator : mcbpmsmparamestlib/Rs Estimator
  Vabc : Outport
  Rs : Outport  Port=2
  Log : Outport  Port=3
  wires:
  Vdc/1 -> Rs Estimator/2
  Config/1 -> Rs Estimator/4
  Rs Estimator/2 -> Rs/1
  StartEst/1 -> Rs Estimator/3
  Rs Estimator/1 -> Vabc/1
  Rs Estimator/3 -> Log/1
  Iabc/1 -> Rs Estimator/1

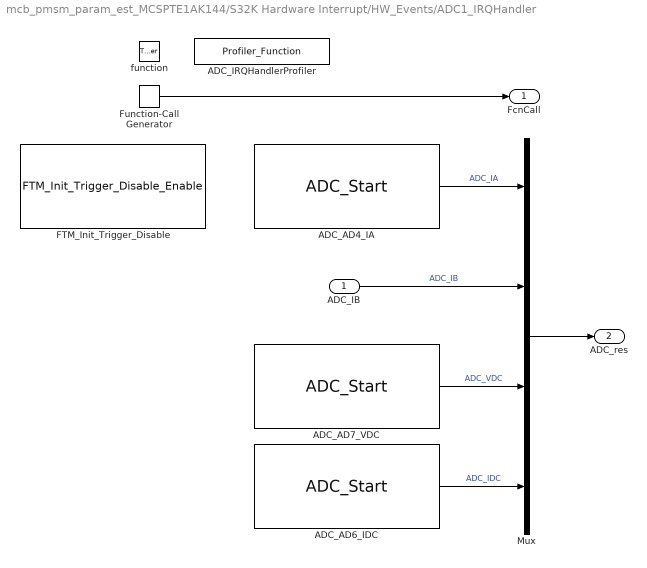
== system mcb_pmsm_param_est_MCSPTE1AK144/S32K Hardware Interrupt/HW_Events/ADC1_IRQHandler ==
  ADC_IB : Inport
  function : TriggerPort  TriggerType=function-call  VariantControl=(inherit)
  ADC_AD4_IA : mbd_s32k1xx_ec_toolbox/Motor Control Blocks/ADC Blocks/ADC_Start  Priority=2  instance=0  adc_r=A  adc_chan=PTB0: [ADC0_SE4 | ADC Single Ended Input]  aien=off  mcuTargetUpdate=on
  ADC_AD6_IDC : mbd_s32k1xx_ec_toolbox/Motor Control Blocks/ADC Blocks/ADC_Start  Priority=4  instance=1  adc_r=B  adc_chan=PTD4: [ADC1_SE6 | ADC Single Ended Input]  aien=off  mcuTargetUpdate=on
  ADC_AD7_VDC : mbd_s32k1xx_ec_toolbox/Motor Control Blocks/ADC Blocks/ADC_Start  Priority=3  instance=1  adc_r=A  adc_chan=PTB12: [ADC1_SE7 | ADC Single Ended Input]  aien=off  mcuTargetUpdate=on
  ADC_IRQHandlerProfiler : mbd_s32k1xx_ec_toolbox/Utility Blocks/Profiler_Function  profile_indx=0
  FTM_Init_Trigger_Disable : mbd_s32k1xx_ec_toolbox/Motor Control Blocks/FTM Blocks/FTM_Init_Trigger_Disable_Enable  Priority=1  ftmModule=3  action=Disable
  Function-Call Generator : simulink/Ports & Subsystems/Function-Call Generator  sample_time=-1  numberOfIterations=1  DisallowWideOutput=off
  Mux : Mux
  FcnCall : Outport  VectorParamsAs1DForOutWhenUnconnected=off
  ADC_res : Outport  Port=2  VectorParamsAs1DForOutWhenUnconnected=off
  wires:
  ADC_AD4_IA/1 -> Mux/1  "ADC_IA"
  ADC_AD7_VDC/1 -> Mux/3  "ADC_VDC"
  Mux/1 -> ADC_res/1
  ADC_AD6_IDC/1 -> Mux/4  "ADC_IDC"
  Function-Call Generator/1 -> FcnCall/1
  ADC_IB/1 -> Mux/2  "ADC_IB"

== system mcb_pmsm_param_est_MCSPTE1AK144/S32K Hardware Interrupt/HW_Events/PDB1_IRQHandler ==
  function : TriggerPort  TriggerType=function-call  VariantControl=(inherit)
  FTM_Init_Trigger_Enable : mbd_s32k1xx_ec_toolbox/Motor Control Blocks/FTM Blocks/FTM_Init_Trigger_Disable_Enable  ftmModule=3  action=Enable

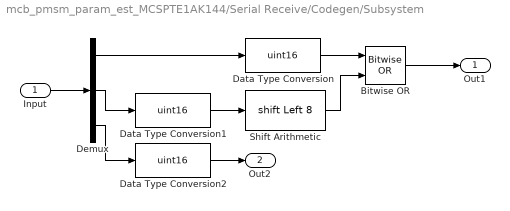
== system mcb_pmsm_param_est_MCSPTE1AK144/Serial Receive/Codegen/Subsystem ==
  Input : Inport  PortDimensions=3
  Bitwise OR : simulink/Logic and Bit Operations/Bitwise Operator  logicop=OR  UseBitMask=off  NumInputPorts=2  BitMask=bin2dec('11011001')  BitMaskRealWorld=Stored Integer
  Data Type Conversion : DataTypeConversion  OutDataTypeStr=uint16  ConvertRealWorld=Stored Integer (SI)  RndMeth=Simplest  SaturateOnIntegerOverflow=off
  Data Type Conversion1 : DataTypeConversion  OutDataTypeStr=uint16  ConvertRealWorld=Stored Integer (SI)  RndMeth=Simplest  SaturateOnIntegerOverflow=off
  Data Type Conversion2 : DataTypeConversion  OutDataTypeStr=uint16  ConvertRealWorld=Stored Integer (SI)  RndMeth=Simplest  SaturateOnIntegerOverflow=off
  Demux : Demux  Outputs=3
  Shift Arithmetic : ArithShift  BitShiftNumber=8  BitShiftDirection=Left
  Out1 : Outport
  Out2 : Outport  Port=2
  wires:
  Data Type Conversion2/1 -> Out2/1
  Shift Arithmetic/1 -> Bitwise OR/2
  Data Type Conversion/1 -> Bitwise OR/1
  Data Type Conversion1/1 -> Shift Arithmetic/1
  Demux/2 -> Data Type Conversion1/1
  Demux/1 -> Data Type Conversion/1
  Bitwise OR/1 -> Out1/1
  Demux/3 -> Data Type Conversion2/1
  Input/1 -> Demux/1

== stateflow chart mcb_pmsm_param_est_MCSPTE1AK144/Hardware Initialization/Enable PDB and start FTM ==
  settings: sampleTime=0.500
  state A
  state END
  (default) -> A
  A -> END : {enablePDB;}
  END -> END : {Normal_Op;}
  events: enablePDB output FUNCTION_CALL_EVENT; Normal_Op output FUNCTION_CALL_EVENT

== stateflow chart mcb_pmsm_param_est_MCSPTE1AK144/Parameter Estimation/Parameter Estimation/Chart ==
  state Init
    during: TestNum = uint16(0);
  state RsTestState
    during: TestNum = uint16(1);
  state LdTestState
    during: TestNum = uint16(2);
  state LqTestState
    during: TestNum = uint16(3);
  state MechTestState
    during: TestNum = uint16(4);
  RsTestState -> Init [order 2] : [EnableIn == 0]
  (default) -> Init
  Init -> RsTestState : [EnableIn == 1 && EnPrev == 0]
  RsTestState -> LdTestState [order 1] : after(1/Ts,tick)[RsStatus == 1]
  MechTestState -> Init : [EnableIn == 0]
  LqTestState -> Init [order 1] : [EnableIn == 0]
  LdTestState -> Init [order 2] : [EnableIn == 0]
  LdTestState -> LqTestState [order 1] : after(1/Ts,tick)[LdStatus == 1]
  LqTestState -> MechTestState [order 2] : after(1/Ts, tick)[LqStatus == 1]
  data: TestNum output; EnableIn input; EnPrev input; RsStatus input; LdStatus input; LqStatus input; Ts input
